simulink model "modulation"  (R2023b)
settings: Solver=VariableStepAuto  StartTime=0.0  StopTime=10.0  RelTol=1e-3
libraries: dspfdesign x2, dspsrcs4 x2
settings Model: Creator=dhanu  LastModifiedBy=dhanu

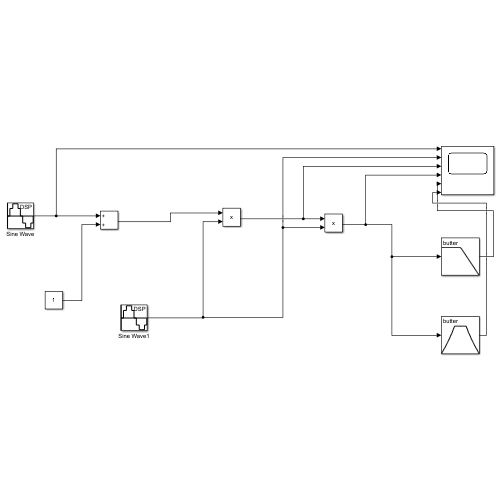
[thumbnail: Simulink's stored preview of the top-level diagram]
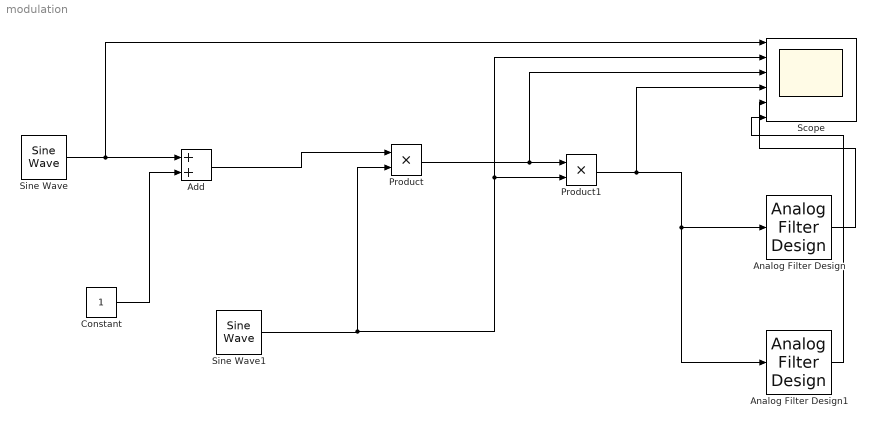
== system modulation ==
  Add : Sum
  Analog Filter Design : dspfdesign/Analog Filter Design  method=Butterworth  filttype=Lowpass  N=20  Wlo=2*3.142*8  Whi=80  Rp=2  Rs=40
  Analog Filter Design1 : dspfdesign/Analog Filter Design  method=Butterworth  filttype=Bandpass  N=20  Wlo=2*3.142*2  Whi=2*3.142*8  Rp=2  Rs=40
  Constant : Constant
  Product : Product
  Product1 : Product
  Scope : Scope  NumInputPorts=6
  Sine Wave : dspsrcs4/Sine Wave  Amplitude=1  Frequency=4  Phase=0  SampleMode=Discrete  OutComplex=Real  CompMethod=Trigonometric fcn  TableSize=Speed  SampleTime=1/500  SamplesPerFrame=1  ResetState=Restart at time zero  OutputFrames=off  dataType=double  wordLen=16  udDataType=sfix(16)  fracBitsMode=Best precision  numFracBits=15  OutDataTypeStr=double  LastOutDataTypeStr=double
  Sine Wave1 : dspsrcs4/Sine Wave  Amplitude=1  Frequency=50  Phase=0  SampleMode=Discrete  OutComplex=Real  CompMethod=Trigonometric fcn  TableSize=Speed  SampleTime=1/5000  SamplesPerFrame=1  ResetState=Restart at time zero  OutputFrames=off  dataType=double  wordLen=16  udDataType=sfix(16)  fracBitsMode=Best precision  numFracBits=15  OutDataTypeStr=double  LastOutDataTypeStr=double
  wires:
  Constant/1 -> Add/2
  Add/1 -> Product/1
  Sine Wave1/1 -> Scope/2, Product1/2, Product/2
  Product/1 -> Scope/3, Product1/1
  Product1/1 -> Scope/4, Analog Filter Design1/1, Analog Filter Design/1
  Sine Wave/1 -> Scope/1, Add/1
  Analog Filter Design/1 -> Scope/5
  Analog Filter Design1/1 -> Scope/6
